simulink model "Utkarsh_2005574_R_W2_P3"  (R2021a)
settings: Solver=VariableStepAuto  StartTime=0.0  StopTime=10.0  RelTol=1e-3
undefined symbols (not defined in the file or in its folder): Ki, Kp, Ts
settings Model: Creator=Utkarsh Anand  LastModifiedBy=Utkarsh Anand

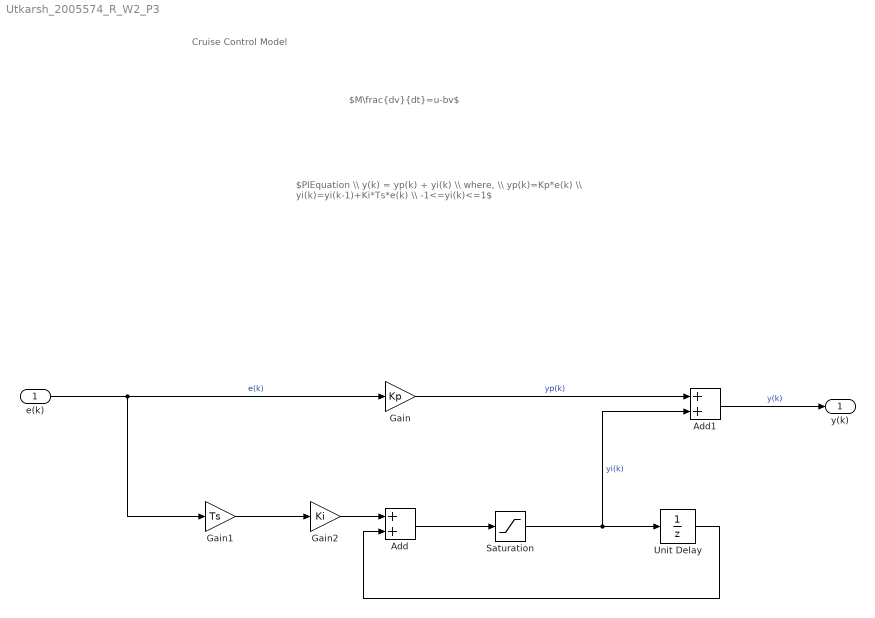
== system Utkarsh_2005574_R_W2_P3 ==
  note: $M\frac{dv}{dt}=u-bv$
  note: Cruise Control Model
  note: $PIEquation \\ y(k) = yp(k) + yi(k) \\ where, \\ yp(k)=Kp*e(k) \\ yi(k)=yi(k-1)+Ki*Ts*e(k) \\ -1<=yi(k)<=1$
  e(k) : Inport  OutDataTypeStr=double  PortDimensions=1  SampleTime=0
  Add : Sum
  Add1 : Sum
  Gain : Gain  Gain=Kp
  Gain1 : Gain  Gain=Ts
  Gain2 : Gain  Gain=Ki
  Saturation : Saturate  UpperLimit=1  LowerLimit=-1
  Unit Delay : UnitDelay  SampleTime=-1  HasFrameUpgradeWarning=on
  y(k) : Outport  OutDataTypeStr=double  PortDimensions=1  SampleTime=0
  wires:
  Add1/1 -> y(k)/1  "y(k)"
  Gain1/1 -> Gain2/1
  Gain/1 -> Add1/1  "yp(k)"
  Unit Delay/1 -> Add/2
  Gain2/1 -> Add/1
  e(k)/1 -> Gain1/1, Gain/1  "e(k)"
  Saturation/1 -> Add1/2, Unit Delay/1  "yi(k)"
  Add/1 -> Saturation/1
